simulink model "modelo"  (R2015a)
settings: Solver=ode45  StartTime=0.0  StopTime=2  RelTol=1e-3
values from neighbouring files (symbols this model uses):
  f1 = 500    [parametros.m]
  fa = 8000    [parametros.m]
  Ta = 1/fa    (= 0.000125)    [parametros.m]
  v1 = 0.2    [parametros.m]
libraries: dspsrcs4 x3, dsparch4 x2
settings Model: Creator=osvaldo.sn  LastModifiedBy=osvaldo.sn

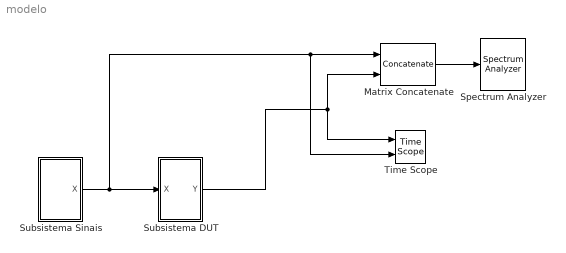
== system modelo ==
  Matrix Concatenate : Concatenate  Mode=Multidimensional array  ConcatenateDimension=2
  Spectrum Analyzer : SpectrumAnalyzer
  Subsistema DUT : Subsystem
  "Subsistema Sinais " : Subsystem
  Time Scope : TimeScope  DefaultConfigurationName=spbscopes.TimeScopeBlockCfg  NumInputPorts=2
  wires:
  "Subsistema Sinais "/1(X) -> Time Scope/2, Matrix Concatenate/1, Subsistema DUT/1(X)
  Subsistema DUT/1(Y) -> Time Scope/1, Matrix Concatenate/2
  Matrix Concatenate/1 -> Spectrum Analyzer/1

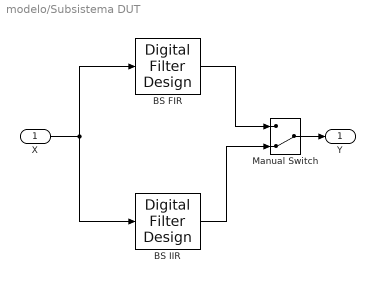
== system modelo/Subsistema DUT ==
  X : Inport
  BS FIR : dsparch4/Digital Filter Design  mwdsp_browser_bugfix_var=off
  BS IIR : dsparch4/Digital Filter Design  mwdsp_browser_bugfix_var=off
  Manual Switch : ManualSwitch  CurrentSetting=0
  Y : Outport
  wires:
  Manual Switch/1 -> Y/1
  BS FIR/1 -> Manual Switch/1
  X/1 -> BS IIR/1, BS FIR/1
  BS IIR/1 -> Manual Switch/2

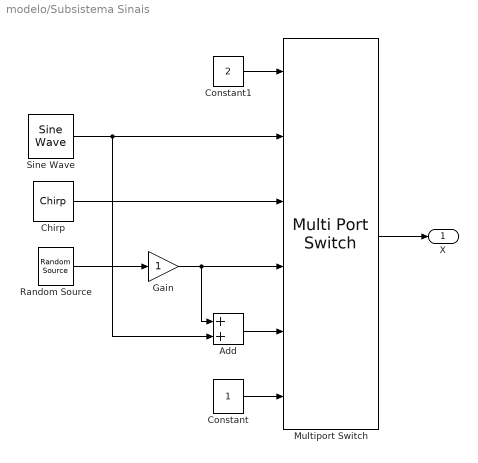
== system modelo/Subsistema Sinais  ==
  Add : Sum
  Chirp : dspsrcs4/Chirp  sweep=Linear  mode=Unidirectional  f0=1  f1=fa/2  t1=2  Tsweep=2  phase=0  Ts=Ta  spf=spf  datatype=Double
  Constant : Constant  VectorParams1D=off
  Constant1 : Constant  Value=2
  Gain : Gain
  Multiport Switch : MultiPortSwitch  Inputs=5
  Random Source : dspsrcs4/Random Source  SrcType=Uniform  NormMethod=Ziggurat  CltLength=12  MinVal=-1  MaxVal=1  MeanVal=0  VarVal=1  RepMode=Not repeatable  rawSeed=1  IsInherit=off  SampMode=Discrete  SampTime=Ta  SampFrame=spf  DataType=Double  OutComplex=Real
  Sine Wave : dspsrcs4/Sine Wave  Amplitude=v1  Frequency=f1  Phase=0  SampleMode=Discrete  OutComplex=Real  CompMethod=Trigonometric fcn  TableSize=Speed  SampleTime=Ta  SamplesPerFrame=spf  ResetState=Restart at time zero  dataType=double  wordLen=16  udDataType=sfix(16)  fracBitsMode=Best precision  numFracBits=15  OutDataTypeStr=double  LastOutDataTypeStr=double
  X : Outport
  wires:
  Constant1/1 -> Multiport Switch/1
  Chirp/1 -> Multiport Switch/3
  Gain/1 -> Add/1, Multiport Switch/4
  Sine Wave/1 -> Multiport Switch/2, Add/2
  Random Source/1 -> Gain/1
  Add/1 -> Multiport Switch/5
  Multiport Switch/1 -> X/1
  Constant/1 -> Multiport Switch/6
